simulink model "simComparacaoEntreAproximacoes"  (R2019b)
settings: Solver=VariableStepAuto  StartTime=0.0  StopTime=10.0  RelTol=1e-3
settings Model: Creator=feliperocha  LastModifiedBy=feliperocha

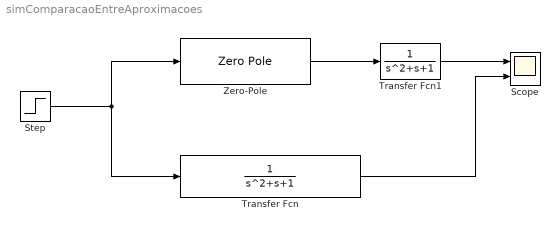
== system simComparacaoEntreAproximacoes ==
  Scope : Scope  NumInputPorts=2
  Step : Step  SampleTime=0
  Transfer Fcn : TransferFcn  Denominator=[1 1 1]
  Transfer Fcn1 : TransferFcn  Denominator=[1 1 1]
  Zero-Pole : ZeroPole  Zeros=[]  Poles=[-.5]  Gain=[.5]
  wires:
  Zero-Pole/1 -> Transfer Fcn1/1
  Step/1 -> Transfer Fcn/1, Zero-Pole/1
  Transfer Fcn/1 -> Scope/2
  Transfer Fcn1/1 -> Scope/1
